simulink model "fsk"  (R2021a)
settings: Solver=FixedStepDiscrete  StartTime=0.0  StopTime=1e-2  FixedStep=1/sampling_freq  RelTol=1e-3
undefined symbols (not defined in the file): coeff, data_rate, nco_1, nco_21, sample_ratio, sampling_freq
libraries: simulink x9, commsink2 x3, commchan3 x2, commdigbbndfm2 x2, commrandsrc2 x1
(part 2 of 2)

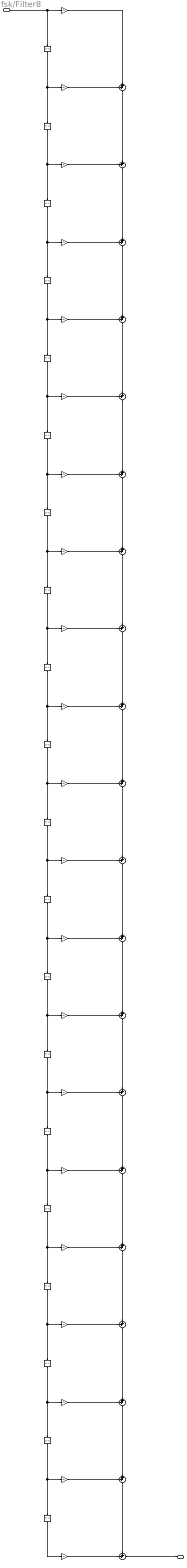
== system fsk/Filter8 ==
  Input : Inport
  BodyDelay{2..21} (20 alike) : Delay  DelayLength=1  InitialCondition=0  InputProcessing=Columns as channels (frame based)
  BodyLSum{2..21} (20 alike) : Sum  Inputs=++|  RndMeth=Nearest  SaturateOnIntegerOverflow=on  OutDataTypeStr=Inherit: Same as first input
  b(1) : Gain  Gain=coeff(1)  ParamDataTypeStr=double  RndMeth=Nearest  SaturateOnIntegerOverflow=on  OutDataTypeStr=Inherit: Same as input
  b(10) : Gain  Gain=coeff(10)  ParamDataTypeStr=double  RndMeth=Nearest  SaturateOnIntegerOverflow=on  OutDataTypeStr=Inherit: Same as input
  b(11) : Gain  Gain=coeff(11)  ParamDataTypeStr=double  RndMeth=Nearest  SaturateOnIntegerOverflow=on  OutDataTypeStr=Inherit: Same as input
  b(12) : Gain  Gain=coeff(12)  ParamDataTypeStr=double  RndMeth=Nearest  SaturateOnIntegerOverflow=on  OutDataTypeStr=Inherit: Same as input
  b(13) : Gain  Gain=coeff(13)  ParamDataTypeStr=double  RndMeth=Nearest  SaturateOnIntegerOverflow=on  OutDataTypeStr=Inherit: Same as input
  b(14) : Gain  Gain=coeff(14)  ParamDataTypeStr=double  RndMeth=Nearest  SaturateOnIntegerOverflow=on  OutDataTypeStr=Inherit: Same as input
  b(15) : Gain  Gain=coeff(15)  ParamDataTypeStr=double  RndMeth=Nearest  SaturateOnIntegerOverflow=on  OutDataTypeStr=Inherit: Same as input
  b(16) : Gain  Gain=coeff(16)  ParamDataTypeStr=double  RndMeth=Nearest  SaturateOnIntegerOverflow=on  OutDataTypeStr=Inherit: Same as input
  b(17) : Gain  Gain=coeff(17)  ParamDataTypeStr=double  RndMeth=Nearest  SaturateOnIntegerOverflow=on  OutDataTypeStr=Inherit: Same as input
  b(18) : Gain  Gain=coeff(18)  ParamDataTypeStr=double  RndMeth=Nearest  SaturateOnIntegerOverflow=on  OutDataTypeStr=Inherit: Same as input
  b(19) : Gain  Gain=coeff(19)  ParamDataTypeStr=double  RndMeth=Nearest  SaturateOnIntegerOverflow=on  OutDataTypeStr=Inherit: Same as input
  b(2) : Gain  Gain=coeff(2)  ParamDataTypeStr=double  RndMeth=Nearest  SaturateOnIntegerOverflow=on  OutDataTypeStr=Inherit: Same as input
  b(20) : Gain  Gain=coeff(20)  ParamDataTypeStr=double  RndMeth=Nearest  SaturateOnIntegerOverflow=on  OutDataTypeStr=Inherit: Same as input
  b(21) : Gain  Gain=coeff(21)  ParamDataTypeStr=double  RndMeth=Nearest  SaturateOnIntegerOverflow=on  OutDataTypeStr=Inherit: Same as input
  b(3) : Gain  Gain=coeff(3)  ParamDataTypeStr=double  RndMeth=Nearest  SaturateOnIntegerOverflow=on  OutDataTypeStr=Inherit: Same as input
  b(4) : Gain  Gain=coeff(4)  ParamDataTypeStr=double  RndMeth=Nearest  SaturateOnIntegerOverflow=on  OutDataTypeStr=Inherit: Same as input
  b(5) : Gain  Gain=coeff(5)  ParamDataTypeStr=double  RndMeth=Nearest  SaturateOnIntegerOverflow=on  OutDataTypeStr=Inherit: Same as input
  b(6) : Gain  Gain=coeff(6)  ParamDataTypeStr=double  RndMeth=Nearest  SaturateOnIntegerOverflow=on  OutDataTypeStr=Inherit: Same as input
  b(7) : Gain  Gain=coeff(7)  ParamDataTypeStr=double  RndMeth=Nearest  SaturateOnIntegerOverflow=on  OutDataTypeStr=Inherit: Same as input
  b(8) : Gain  Gain=coeff(8)  ParamDataTypeStr=double  RndMeth=Nearest  SaturateOnIntegerOverflow=on  OutDataTypeStr=Inherit: Same as input
  b(9) : Gain  Gain=coeff(9)  ParamDataTypeStr=double  RndMeth=Nearest  SaturateOnIntegerOverflow=on  OutDataTypeStr=Inherit: Same as input
  Output : Outport
  wires:
  Input/1 -> b(1)/1, BodyDelay2/1
  b(1)/1 -> BodyLSum2/2
  BodyDelay2/1 -> b(2)/1, BodyDelay3/1
  b(2)/1 -> BodyLSum2/1
  BodyLSum2/1 -> BodyLSum3/2
  BodyDelay3/1 -> b(3)/1, BodyDelay4/1
  b(3)/1 -> BodyLSum3/1
  BodyLSum3/1 -> BodyLSum4/2
  BodyDelay4/1 -> b(4)/1, BodyDelay5/1
  b(4)/1 -> BodyLSum4/1
  BodyLSum4/1 -> BodyLSum5/2
  BodyDelay5/1 -> b(5)/1, BodyDelay6/1
  b(5)/1 -> BodyLSum5/1
  BodyLSum5/1 -> BodyLSum6/2
  BodyDelay6/1 -> b(6)/1, BodyDelay7/1
  b(6)/1 -> BodyLSum6/1
  BodyLSum6/1 -> BodyLSum7/2
  BodyDelay7/1 -> b(7)/1, BodyDelay8/1
  b(7)/1 -> BodyLSum7/1
  BodyLSum7/1 -> BodyLSum8/2
  BodyDelay8/1 -> b(8)/1, BodyDelay9/1
  b(8)/1 -> BodyLSum8/1
  BodyLSum8/1 -> BodyLSum9/2
  BodyDelay9/1 -> b(9)/1, BodyDelay10/1
  b(9)/1 -> BodyLSum9/1
  BodyLSum9/1 -> BodyLSum10/2
  BodyDelay10/1 -> b(10)/1, BodyDelay11/1
  b(10)/1 -> BodyLSum10/1
  BodyLSum10/1 -> BodyLSum11/2
  BodyDelay11/1 -> b(11)/1, BodyDelay12/1
  b(11)/1 -> BodyLSum11/1
  BodyLSum11/1 -> BodyLSum12/2
  BodyDelay12/1 -> b(12)/1, BodyDelay13/1
  b(12)/1 -> BodyLSum12/1
  BodyLSum12/1 -> BodyLSum13/2
  BodyDelay13/1 -> b(13)/1, BodyDelay14/1
  b(13)/1 -> BodyLSum13/1
  BodyLSum13/1 -> BodyLSum14/2
  BodyDelay14/1 -> b(14)/1, BodyDelay15/1
  b(14)/1 -> BodyLSum14/1
  BodyLSum14/1 -> BodyLSum15/2
  BodyDelay15/1 -> b(15)/1, BodyDelay16/1
  b(15)/1 -> BodyLSum15/1
  BodyLSum15/1 -> BodyLSum16/2
  BodyDelay16/1 -> b(16)/1, BodyDelay17/1
  b(16)/1 -> BodyLSum16/1
  BodyLSum16/1 -> BodyLSum17/2
  BodyDelay17/1 -> b(17)/1, BodyDelay18/1
  b(17)/1 -> BodyLSum17/1
  BodyLSum17/1 -> BodyLSum18/2
  BodyDelay18/1 -> b(18)/1, BodyDelay19/1
  b(18)/1 -> BodyLSum18/1
  BodyLSum18/1 -> BodyLSum19/2
  BodyDelay19/1 -> b(19)/1, BodyDelay20/1
  b(19)/1 -> BodyLSum19/1
  BodyLSum19/1 -> BodyLSum20/2
  BodyDelay20/1 -> b(20)/1, BodyDelay21/1
  b(20)/1 -> BodyLSum20/1
  BodyLSum20/1 -> BodyLSum21/1
  BodyDelay21/1 -> b(21)/1
  b(21)/1 -> BodyLSum21/2
  BodyLSum21/1 -> Output/1

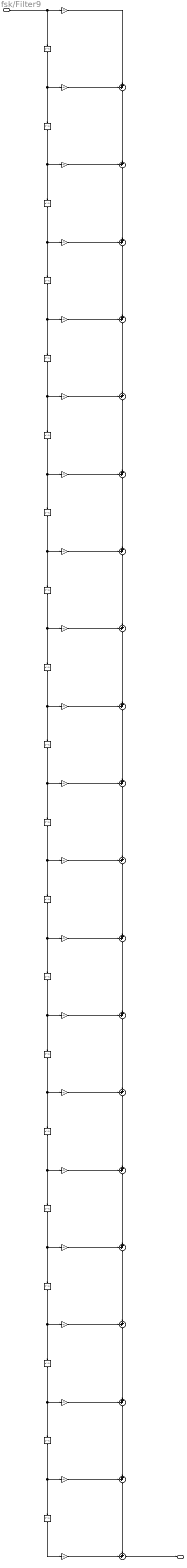
== system fsk/Filter9 ==
  Input : Inport
  BodyDelay{2..21} (20 alike) : Delay  DelayLength=1  InitialCondition=0  InputProcessing=Columns as channels (frame based)
  BodyLSum{2..21} (20 alike) : Sum  Inputs=++|  RndMeth=Nearest  SaturateOnIntegerOverflow=on  OutDataTypeStr=Inherit: Same as first input
  b(1) : Gain  Gain=coeff(1)  ParamDataTypeStr=double  RndMeth=Nearest  SaturateOnIntegerOverflow=on  OutDataTypeStr=Inherit: Same as input
  b(10) : Gain  Gain=coeff(10)  ParamDataTypeStr=double  RndMeth=Nearest  SaturateOnIntegerOverflow=on  OutDataTypeStr=Inherit: Same as input
  b(11) : Gain  Gain=coeff(11)  ParamDataTypeStr=double  RndMeth=Nearest  SaturateOnIntegerOverflow=on  OutDataTypeStr=Inherit: Same as input
  b(12) : Gain  Gain=coeff(12)  ParamDataTypeStr=double  RndMeth=Nearest  SaturateOnIntegerOverflow=on  OutDataTypeStr=Inherit: Same as input
  b(13) : Gain  Gain=coeff(13)  ParamDataTypeStr=double  RndMeth=Nearest  SaturateOnIntegerOverflow=on  OutDataTypeStr=Inherit: Same as input
  b(14) : Gain  Gain=coeff(14)  ParamDataTypeStr=double  RndMeth=Nearest  SaturateOnIntegerOverflow=on  OutDataTypeStr=Inherit: Same as input
  b(15) : Gain  Gain=coeff(15)  ParamDataTypeStr=double  RndMeth=Nearest  SaturateOnIntegerOverflow=on  OutDataTypeStr=Inherit: Same as input
  b(16) : Gain  Gain=coeff(16)  ParamDataTypeStr=double  RndMeth=Nearest  SaturateOnIntegerOverflow=on  OutDataTypeStr=Inherit: Same as input
  b(17) : Gain  Gain=coeff(17)  ParamDataTypeStr=double  RndMeth=Nearest  SaturateOnIntegerOverflow=on  OutDataTypeStr=Inherit: Same as input
  b(18) : Gain  Gain=coeff(18)  ParamDataTypeStr=double  RndMeth=Nearest  SaturateOnIntegerOverflow=on  OutDataTypeStr=Inherit: Same as input
  b(19) : Gain  Gain=coeff(19)  ParamDataTypeStr=double  RndMeth=Nearest  SaturateOnIntegerOverflow=on  OutDataTypeStr=Inherit: Same as input
  b(2) : Gain  Gain=coeff(2)  ParamDataTypeStr=double  RndMeth=Nearest  SaturateOnIntegerOverflow=on  OutDataTypeStr=Inherit: Same as input
  b(20) : Gain  Gain=coeff(20)  ParamDataTypeStr=double  RndMeth=Nearest  SaturateOnIntegerOverflow=on  OutDataTypeStr=Inherit: Same as input
  b(21) : Gain  Gain=coeff(21)  ParamDataTypeStr=double  RndMeth=Nearest  SaturateOnIntegerOverflow=on  OutDataTypeStr=Inherit: Same as input
  b(3) : Gain  Gain=coeff(3)  ParamDataTypeStr=double  RndMeth=Nearest  SaturateOnIntegerOverflow=on  OutDataTypeStr=Inherit: Same as input
  b(4) : Gain  Gain=coeff(4)  ParamDataTypeStr=double  RndMeth=Nearest  SaturateOnIntegerOverflow=on  OutDataTypeStr=Inherit: Same as input
  b(5) : Gain  Gain=coeff(5)  ParamDataTypeStr=double  RndMeth=Nearest  SaturateOnIntegerOverflow=on  OutDataTypeStr=Inherit: Same as input
  b(6) : Gain  Gain=coeff(6)  ParamDataTypeStr=double  RndMeth=Nearest  SaturateOnIntegerOverflow=on  OutDataTypeStr=Inherit: Same as input
  b(7) : Gain  Gain=coeff(7)  ParamDataTypeStr=double  RndMeth=Nearest  SaturateOnIntegerOverflow=on  OutDataTypeStr=Inherit: Same as input
  b(8) : Gain  Gain=coeff(8)  ParamDataTypeStr=double  RndMeth=Nearest  SaturateOnIntegerOverflow=on  OutDataTypeStr=Inherit: Same as input
  b(9) : Gain  Gain=coeff(9)  ParamDataTypeStr=double  RndMeth=Nearest  SaturateOnIntegerOverflow=on  OutDataTypeStr=Inherit: Same as input
  Output : Outport
  wires:
  Input/1 -> b(1)/1, BodyDelay2/1
  b(1)/1 -> BodyLSum2/2
  BodyDelay2/1 -> b(2)/1, BodyDelay3/1
  b(2)/1 -> BodyLSum2/1
  BodyLSum2/1 -> BodyLSum3/2
  BodyDelay3/1 -> b(3)/1, BodyDelay4/1
  b(3)/1 -> BodyLSum3/1
  BodyLSum3/1 -> BodyLSum4/2
  BodyDelay4/1 -> b(4)/1, BodyDelay5/1
  b(4)/1 -> BodyLSum4/1
  BodyLSum4/1 -> BodyLSum5/2
  BodyDelay5/1 -> b(5)/1, BodyDelay6/1
  b(5)/1 -> BodyLSum5/1
  BodyLSum5/1 -> BodyLSum6/2
  BodyDelay6/1 -> b(6)/1, BodyDelay7/1
  b(6)/1 -> BodyLSum6/1
  BodyLSum6/1 -> BodyLSum7/2
  BodyDelay7/1 -> b(7)/1, BodyDelay8/1
  b(7)/1 -> BodyLSum7/1
  BodyLSum7/1 -> BodyLSum8/2
  BodyDelay8/1 -> b(8)/1, BodyDelay9/1
  b(8)/1 -> BodyLSum8/1
  BodyLSum8/1 -> BodyLSum9/2
  BodyDelay9/1 -> b(9)/1, BodyDelay10/1
  b(9)/1 -> BodyLSum9/1
  BodyLSum9/1 -> BodyLSum10/2
  BodyDelay10/1 -> b(10)/1, BodyDelay11/1
  b(10)/1 -> BodyLSum10/1
  BodyLSum10/1 -> BodyLSum11/2
  BodyDelay11/1 -> b(11)/1, BodyDelay12/1
  b(11)/1 -> BodyLSum11/1
  BodyLSum11/1 -> BodyLSum12/2
  BodyDelay12/1 -> b(12)/1, BodyDelay13/1
  b(12)/1 -> BodyLSum12/1
  BodyLSum12/1 -> BodyLSum13/2
  BodyDelay13/1 -> b(13)/1, BodyDelay14/1
  b(13)/1 -> BodyLSum13/1
  BodyLSum13/1 -> BodyLSum14/2
  BodyDelay14/1 -> b(14)/1, BodyDelay15/1
  b(14)/1 -> BodyLSum14/1
  BodyLSum14/1 -> BodyLSum15/2
  BodyDelay15/1 -> b(15)/1, BodyDelay16/1
  b(15)/1 -> BodyLSum15/1
  BodyLSum15/1 -> BodyLSum16/2
  BodyDelay16/1 -> b(16)/1, BodyDelay17/1
  b(16)/1 -> BodyLSum16/1
  BodyLSum16/1 -> BodyLSum17/2
  BodyDelay17/1 -> b(17)/1, BodyDelay18/1
  b(17)/1 -> BodyLSum17/1
  BodyLSum17/1 -> BodyLSum18/2
  BodyDelay18/1 -> b(18)/1, BodyDelay19/1
  b(18)/1 -> BodyLSum18/1
  BodyLSum18/1 -> BodyLSum19/2
  BodyDelay19/1 -> b(19)/1, BodyDelay20/1
  b(19)/1 -> BodyLSum19/1
  BodyLSum19/1 -> BodyLSum20/2
  BodyDelay20/1 -> b(20)/1, BodyDelay21/1
  b(20)/1 -> BodyLSum20/1
  BodyLSum20/1 -> BodyLSum21/1
  BodyDelay21/1 -> b(21)/1
  b(21)/1 -> BodyLSum21/2
  BodyLSum21/1 -> Output/1

== system fsk/NCO ==
  Add : Sum  AccumDataTypeStr=double
  Constant : Constant  Value=nco_21  OutDataTypeStr=double  SampleTime=1/sampling_freq
  Data Type Conversion : DataTypeConversion  OutMin=[0]  OutMax=[2]  OutDataTypeStr=fixdt(0,8)
  Delay1 : Delay  DelayLength=1  InitialCondition=0  UseCircularBuffer=on  SampleTime=1/sampling_freq
  Sine Lookup : simulink/Lookup Tables/Sine  Formula=sin(2*pi*u)  NumDataPoints=(2^3)+1  OutputWordLength=8  InternalRulePriority=Speed
  Out1 : Outport
  wires:
  Delay1/1 -> Add/2
  Constant/1 -> Add/1
  Add/1 -> Delay1/1, Data Type Conversion/1
  Data Type Conversion/1 -> Sine Lookup/1
  Sine Lookup/1 -> Out1/1

== system fsk/NCO1 ==
  Add : Sum  AccumDataTypeStr=double
  Constant : Constant  Value=nco_21/2  OutDataTypeStr=double  SampleTime=1/sampling_freq
  Data Type Conversion : DataTypeConversion  OutMin=[0]  OutMax=[2]  OutDataTypeStr=fixdt(0,8)
  Delay1 : Delay  DelayLength=1  InitialCondition=0  UseCircularBuffer=on  SampleTime=1/sampling_freq
  Sine Lookup : simulink/Lookup Tables/Sine  Formula=sin(2*pi*u)  NumDataPoints=(2^3)+1  OutputWordLength=8  InternalRulePriority=Speed
  Out1 : Outport
  wires:
  Sine Lookup/1 -> Out1/1
  Delay1/1 -> Add/2
  Constant/1 -> Add/1
  Add/1 -> Delay1/1, Data Type Conversion/1
  Data Type Conversion/1 -> Sine Lookup/1

== system fsk/NCO2 ==
  Add : Sum  AccumDataTypeStr=double
  Constant : Constant  Value=nco_21  OutDataTypeStr=double  SampleTime=1/sampling_freq
  Data Type Conversion : DataTypeConversion  OutMin=[0]  OutMax=[2]  OutDataTypeStr=fixdt(0,8)
  Delay1 : Delay  DelayLength=1  InitialCondition=0  UseCircularBuffer=on  SampleTime=1/sampling_freq
  Sine Lookup : simulink/Lookup Tables/Sine  Formula=sin(2*pi*u)  NumDataPoints=(2^3)+1  OutputWordLength=8  InternalRulePriority=Speed
  Out1 : Outport
  wires:
  Sine Lookup/1 -> Out1/1
  Delay1/1 -> Add/2
  Constant/1 -> Add/1
  Add/1 -> Delay1/1, Data Type Conversion/1
  Data Type Conversion/1 -> Sine Lookup/1

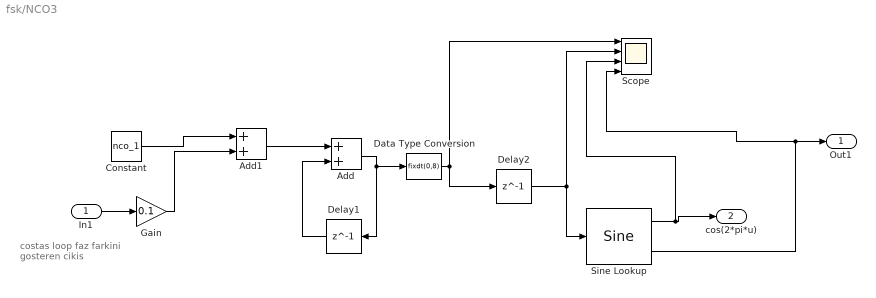
== system fsk/NCO3 ==
  note: costas loop faz farkini gosteren cikis
  In1 : Inport
  Add : Sum  AccumDataTypeStr=double
  Add1 : Sum
  Constant : Constant  Value=nco_1  OutDataTypeStr=double  SampleTime=1/sampling_freq
  Data Type Conversion : DataTypeConversion  OutMin=[0]  OutMax=[2]  OutDataTypeStr=fixdt(0,8)
  Delay1 : Delay  DelayLength=1  InitialCondition=0  UseCircularBuffer=on  SampleTime=1/sampling_freq
  Delay2 : Delay  DelayLength=1  InitialCondition=0  UseCircularBuffer=on  SampleTime=1/sampling_freq
  Gain : Gain  Gain=0.1
  Scope : Scope  NumInputPorts=4
  Sine Lookup : simulink/Lookup Tables/Sine  Formula=sin(2*pi*u) and cos(2*pi*u)  NumDataPoints=(2^2)+1  OutputWordLength=8  InternalRulePriority=Speed
  Out1 : Outport
  cos(2*pi*u) : Outport  Port=2
  wires:
  Sine Lookup/2 -> Scope/4, Out1/1
  Sine Lookup/1 -> Scope/3, cos(2*pi*u)/1
  Delay1/1 -> Add/2
  Add/1 -> Delay1/1, Data Type Conversion/1
  Data Type Conversion/1 -> Delay2/1, Scope/1
  Add1/1 -> Add/1
  Constant/1 -> Add1/1
  Gain/1 -> Add1/2
  In1/1 -> Gain/1
  Delay2/1 -> Scope/2, Sine Lookup/1

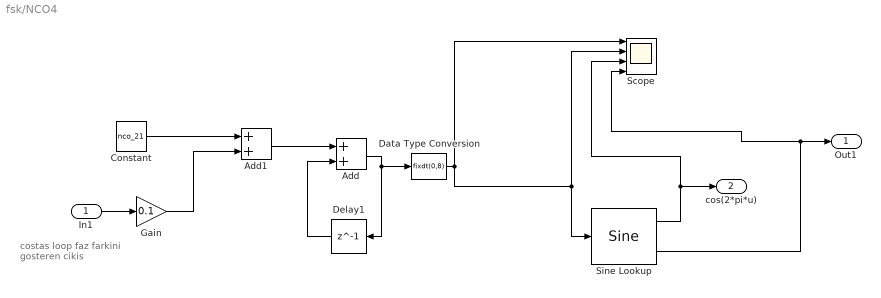
== system fsk/NCO4 ==
  note: costas loop faz farkini gosteren cikis
  In1 : Inport
  Add : Sum  AccumDataTypeStr=double
  Add1 : Sum
  Constant : Constant  Value=nco_21  OutDataTypeStr=double  SampleTime=1/sampling_freq
  Data Type Conversion : DataTypeConversion  OutMin=[0]  OutMax=[2]  OutDataTypeStr=fixdt(0,8)
  Delay1 : Delay  DelayLength=1  InitialCondition=0  UseCircularBuffer=on  SampleTime=1/sampling_freq
  Gain : Gain  Gain=0.1
  Scope : Scope  NumInputPorts=4
  Sine Lookup : simulink/Lookup Tables/Sine  Formula=sin(2*pi*u) and cos(2*pi*u)  NumDataPoints=(2^3)+1  OutputWordLength=8  InternalRulePriority=Speed
  Out1 : Outport
  cos(2*pi*u) : Outport  Port=2
  wires:
  Sine Lookup/2 -> Scope/4, Out1/1
  Sine Lookup/1 -> Scope/3, cos(2*pi*u)/1
  Delay1/1 -> Add/2
  Add/1 -> Delay1/1, Data Type Conversion/1
  Add1/1 -> Add/1
  Constant/1 -> Add1/1
  In1/1 -> Gain/1
  Gain/1 -> Add1/2
  Data Type Conversion/1 -> Scope/2, Sine Lookup/1, Scope/1

== system fsk/NCO5 ==
  Add : Sum  AccumDataTypeStr=double
  Constant : Constant  Value=nco_1  OutDataTypeStr=double  SampleTime=25e-9
  Data Type Conversion : DataTypeConversion  OutMin=[0]  OutMax=[2]  OutDataTypeStr=fixdt(0,8)
  Delay1 : Delay  DelayLength=1  InitialCondition=0  UseCircularBuffer=on  SampleTime=1/sampling_freq
  Scope : Scope  NumInputPorts=4
  Sine Lookup : simulink/Lookup Tables/Sine  Formula=sin(2*pi*u) and cos(2*pi*u)  NumDataPoints=(2^2)+1  OutputWordLength=8  InternalRulePriority=Speed
  Out2 : Outport
  wires:
  Sine Lookup/2 -> Scope/4
  Sine Lookup/1 -> Out2/1, Scope/3
  Delay1/1 -> Add/2
  Constant/1 -> Add/1
  Add/1 -> Delay1/1, Data Type Conversion/1
  Data Type Conversion/1 -> Scope/2, Sine Lookup/1, Scope/1

== system fsk/NCO6 ==
  note: costas loop faz farkini gosteren cikis
  In1 : Inport
  Add : Sum  AccumDataTypeStr=double
  Add1 : Sum
  Constant : Constant  Value=nco_21  OutDataTypeStr=double  SampleTime=1/sampling_freq
  Data Type Conversion : DataTypeConversion  OutMin=[0]  OutMax=[2]  OutDataTypeStr=fixdt(0,8)
  Delay1 : Delay  DelayLength=1  InitialCondition=0  UseCircularBuffer=on  SampleTime=1/sampling_freq
  Gain : Gain  Gain=0.1
  Sine Lookup : simulink/Lookup Tables/Sine  Formula=sin(2*pi*u) and cos(2*pi*u)  NumDataPoints=(2^3)+1  OutputWordLength=8  InternalRulePriority=Speed
  Out1 : Outport
  sin(2*pi*u) : Outport  Port=2
  wires:
  Sine Lookup/2 -> Out1/1
  Sine Lookup/1 -> sin(2*pi*u)/1
  Delay1/1 -> Add/2
  Add/1 -> Delay1/1, Data Type Conversion/1
  Add1/1 -> Add/1
  Constant/1 -> Add1/1
  Gain/1 -> Add1/2
  In1/1 -> Gain/1
  Data Type Conversion/1 -> Sine Lookup/1
